simulink model "d2"  (R2025a)
settings: Solver=VariableStepAuto  StartTime=0.0  StopTime=100  RelTol=1e-3
settings Model: Creator=Korisnik  LastModifiedBy=Korisnik

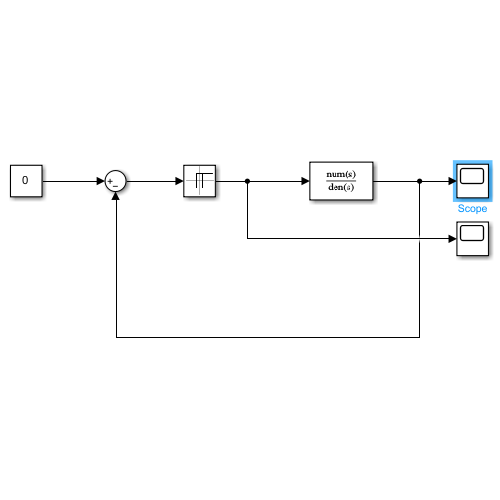
[thumbnail: Simulink's stored preview of the top-level diagram]
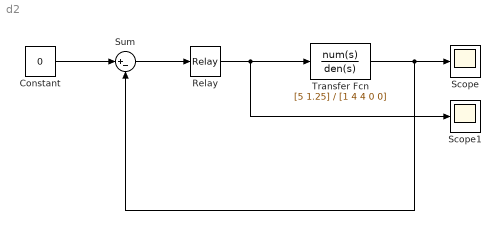
== system d2 ==
  Constant : Constant  Value=0
  Relay : Relay  OnSwitchValue=0.1  OffSwitchValue=-0.1  OffOutputValue=-1
  Scope : Scope
      settings: ActiveDisplayYMinimum=-0.47478028608834283  ActiveDisplayYMaximum=0.4002692714766653
  Scope1 : Scope
      settings: ActiveDisplayYMinimum=-0.73697413400932754  ActiveDisplayYMaximum=0.31886120611056612
  Sum : Sum  Inputs=|+-
  Transfer Fcn : TransferFcn  Numerator=[5 1.25]  Denominator=[1 4 4 0 0]
  wires:
  Transfer Fcn/1 -> Sum/2, Scope/1
  Constant/1 -> Sum/1
  Sum/1 -> Relay/1
  Relay/1 -> Scope1/1, Transfer Fcn/1
